simulink model "M005_refor_control"  (R2021a)
settings: Solver=VariableStepAuto  StartTime=0.0  StopTime=30  RelTol=1e-3
settings Model: Creator=djoroya  LastModifiedBy=djoroya

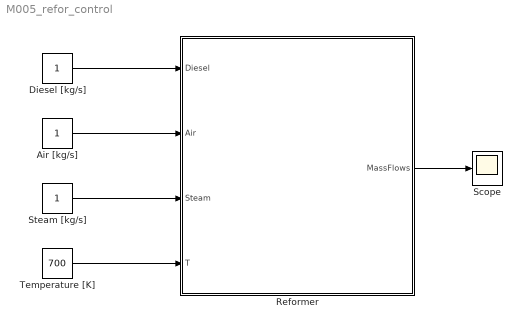
== system M005_refor_control ==
  Air [kg/s] : Constant
  Diesel [kg/s] : Constant
  "Reformer " : Subsystem
  Scope : Scope
  Steam [kg/s] : Constant
  Temperature [K] : Constant  Value=700
  wires:
  Diesel [kg/s]/1 -> "Reformer "/1(Diesel)
  Air [kg/s]/1 -> "Reformer "/2(Air)
  Steam [kg/s]/1 -> "Reformer "/3(Steam)
  Temperature [K]/1 -> "Reformer "/4(T)
  "Reformer "/1(MassFlows) -> Scope/1

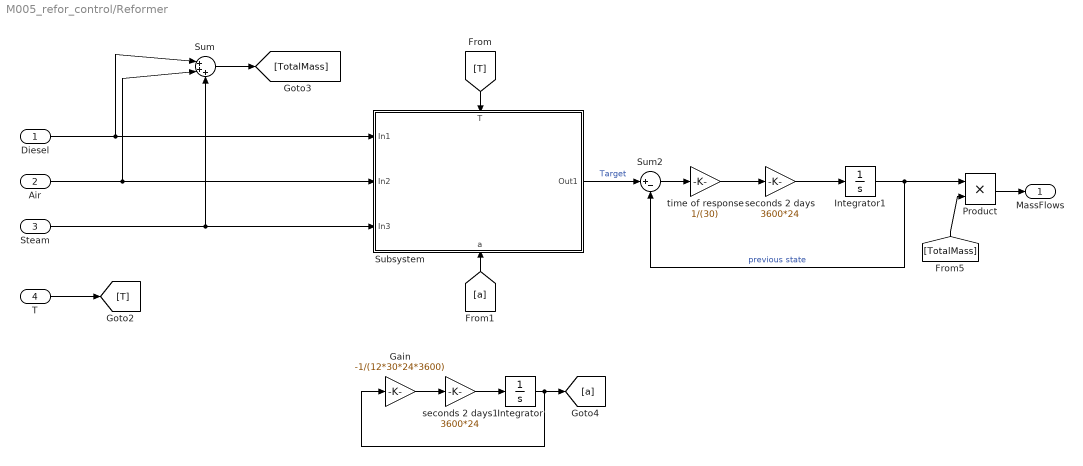
== system M005_refor_control/Reformer  ==
  Diesel : Inport
  Air : Inport  Port=2
  Steam : Inport  Port=3
  T : Inport  Port=4
  Gain : Gain  Gain=-1/(12*30*24*3600)
  Integrator : Integrator  InitialCondition=1
  Integrator1 : Integrator
  Product : Product
  Subsystem : Subsystem
      settings: PortSchema="{\"entries\":[{\"content\":{\"sides\":[{\"content\":{\"connectorIds\":[\"In1\",\"In2\",\"In3\"]},\"type\":\"ConnectorPlacement.EquallySpacedRectSide\",\"uuid\":\"0dada652-6957-4c3e-8e48-73ee360a3bab\"},{\"content\":{\"connectorIds\":[\"Out1\"],\"side\":\"RIGHT\"},\"type\":\"ConnectorPlacement.EquallySpacedRectSide\",\"uuid\":\"81208621-951c-43f9-b655-3502a16ce57a\"},{\"content\":{\"connectorIds\":[\"In4\"],\"side\":\"TOP\"},\"type\":\"ConnectorPlacement.EquallySpacedRectSide\",\"uuid\":\"1012e2be-7d0b-44a9-9a40-bc453950010e\"},{\"content\":{\"connectorIds\":[\"In5\"],\"side\":\"BOTTOM\"},\"type\":\"ConnectorPlacement.EquallySpacedRectSide\",\"uuid\":\"aaef83a2-abb7-4780-82b5-9abad57d39ad\"}]},\"type\":\"ConnectorPlacement.EquallySpacedConnector\",\"uuid\":\"1143871f-aacc-4fa7-a444-9910d5016eff\"}],\"packageUris\":[\"http://schema.mathworks.com/mf0/Connector/R2020b\"],\"version\":\"1.0\"}"
  Sum : Sum  Inputs=|+++
  Sum2 : Sum  Inputs=|+-
  seconds 2 days : Gain  Gain=3600*24
  seconds 2 days1 : Gain  Gain=3600*24
  time of response : Gain  Gain=1/(30)
  MassFlows : Outport
  wires:
  Product/1 -> MassFlows/1
  T/1 -> [T]
  Sum/1 -> [TotalMass]
  Integrator/1 -> Gain/1, [a]
  [TotalMass] -> Product/2
  Steam/1 -> Sum/3, Subsystem/3(In3)
  Diesel/1 -> Sum/1, Subsystem/1(In1)
  Air/1 -> Sum/2, Subsystem/2(In2)
  seconds 2 days1/1 -> Integrator/1
  Gain/1 -> seconds 2 days1/1
  [a] -> Subsystem/5(a)
  [T] -> Subsystem/4(T)
  seconds 2 days/1 -> Integrator1/1
  Subsystem/1(Out1) -> Sum2/1  "Target"
  time of response/1 -> seconds 2 days/1
  Integrator1/1 -> Product/1, Sum2/2  "previous state"
  Sum2/1 -> time of response/1

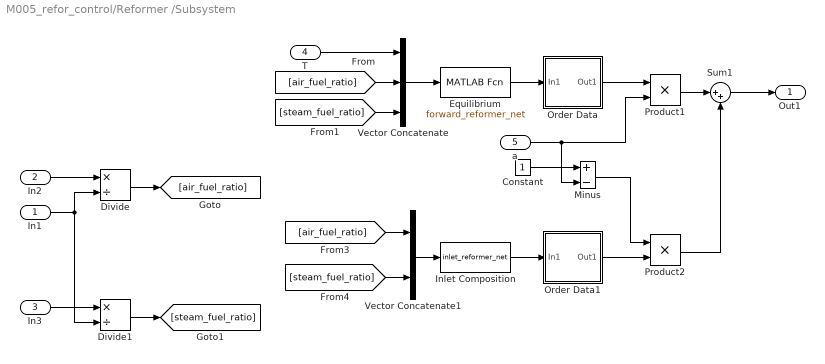
== system M005_refor_control/Reformer /Subsystem ==
  In1 : Inport
  In2 : Inport  Port=2
  In3 : Inport  Port=3
  T : Inport  Port=4
  a : Inport  Port=5
  Constant : Constant
  Divide : Product  Inputs=*/
  Divide1 : Product  Inputs=*/
  Equilibrium : MATLABFcn  MATLABFcn=forward_reformer_net  OutputDimensions=8  OutputSignalType=real  Output1D=off
  Inlet Composition : MATLABFcn  MATLABFcn=inlet_reformer_net  OutputDimensions=6  OutputSignalType=real  Output1D=off
  Minus : Sum  Inputs=+-
  Order Data : Subsystem
  Order Data1 : Subsystem
  Product1 : Product
  Product2 : Product
  Sum1 : Sum  Inputs=|++
  Vector Concatenate : Concatenate  NumInputs=3
  Vector Concatenate1 : Concatenate
  Out1 : Outport
  wires:
  a/1 -> Product1/2, Minus/2
  [steam_fuel_ratio] -> Vector Concatenate/3
  In2/1 -> Divide/1
  Product1/1 -> Sum1/1
  T/1 -> Vector Concatenate/1
  [air_fuel_ratio] -> Vector Concatenate1/1
  Vector Concatenate/1 -> Equilibrium/1
  Product2/1 -> Sum1/2
  [steam_fuel_ratio] -> Vector Concatenate1/2
  Divide/1 -> [air_fuel_ratio]
  Order Data1/1(Out1) -> Product2/2
  Minus/1 -> Product2/1
  Divide1/1 -> [steam_fuel_ratio]
  Inlet Composition/1 -> Order Data1/1(In1)
  Order Data/1(Out1) -> Product1/1
  Vector Concatenate1/1 -> Inlet Composition/1
  [air_fuel_ratio] -> Vector Concatenate/2
  Equilibrium/1 -> Order Data/1(In1)
  Constant/1 -> Minus/1
  In3/1 -> Divide1/1
  In1/1 -> Divide/2, Divide1/2
  Sum1/1 -> Out1/1

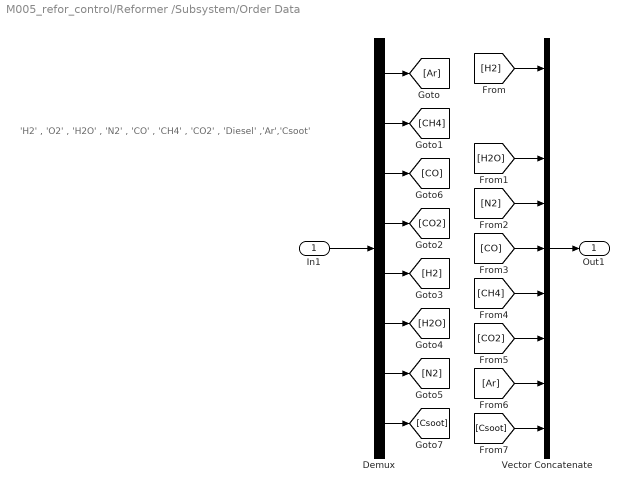
== system M005_refor_control/Reformer /Subsystem/Order Data ==
  note: 'H2' , 'O2' , 'H2O' , 'N2' , 'CO' , 'CH4' , 'CO2' , 'Diesel' ,'Ar','Csoot'
  In1 : Inport
  Demux : Demux  Outputs=8
  Vector Concatenate : Concatenate  NumInputs=9
  Out1 : Outport
  wires:
  In1/1 -> Demux/1
  Demux/1 -> [Ar]
  Demux/2 -> [CH4]
  Demux/3 -> [CO]
  Demux/4 -> [CO2]
  Demux/5 -> [H2]
  Demux/6 -> [H2O]
  Demux/7 -> [N2]
  Demux/8 -> [Csoot]
  [H2] -> Vector Concatenate/1
  [H2O] -> Vector Concatenate/3
  [N2] -> Vector Concatenate/4
  [CO] -> Vector Concatenate/5
  [CH4] -> Vector Concatenate/6
  [CO2] -> Vector Concatenate/7
  [Ar] -> Vector Concatenate/8
  [Csoot] -> Vector Concatenate/9
  Vector Concatenate/1 -> Out1/1

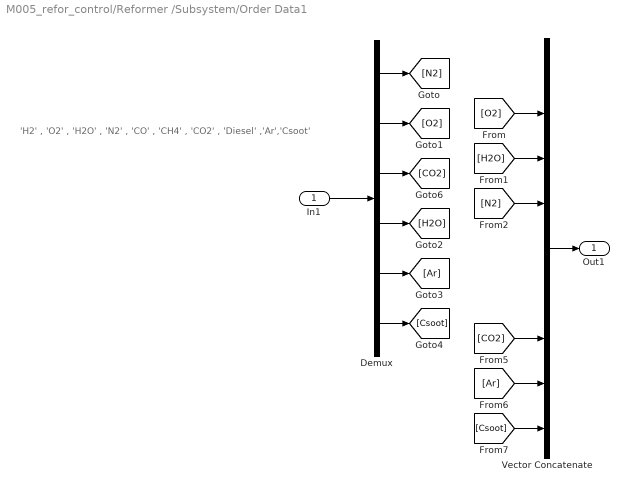
== system M005_refor_control/Reformer /Subsystem/Order Data1 ==
  note: 'H2' , 'O2' , 'H2O' , 'N2' , 'CO' , 'CH4' , 'CO2' , 'Diesel' ,'Ar','Csoot'
  In1 : Inport
  Demux : Demux  Outputs=6
  Vector Concatenate : Concatenate  NumInputs=9
  Out1 : Outport
  wires:
  In1/1 -> Demux/1
  Demux/1 -> [N2]
  Demux/2 -> [O2]
  Demux/3 -> [CO2]
  Demux/4 -> [H2O]
  Demux/5 -> [Ar]
  Demux/6 -> [Csoot]
  [H2O] -> Vector Concatenate/3
  [N2] -> Vector Concatenate/4
  [CO2] -> Vector Concatenate/7
  [Ar] -> Vector Concatenate/8
  [Csoot] -> Vector Concatenate/9
  Vector Concatenate/1 -> Out1/1
  [O2] -> Vector Concatenate/2
